simulink model "sudarshan_simulink3"  (R2021b)
settings: Solver=VariableStepAuto  StartTime=0.0  StopTime=0.01  RelTol=1e-3
settings Model: Creator=year2  LastModifiedBy=year2

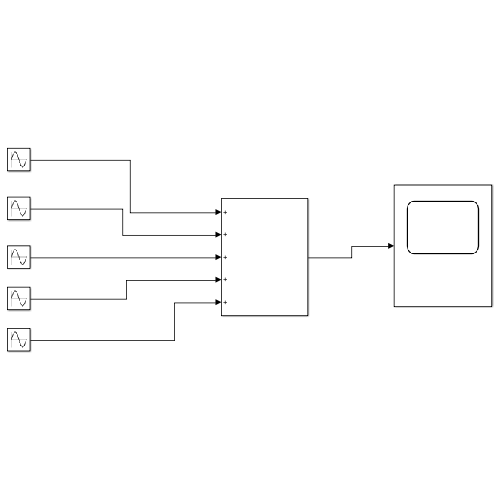
[thumbnail: Simulink's stored preview of the top-level diagram]
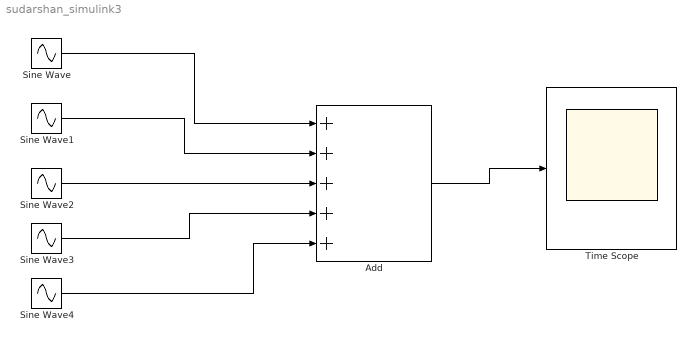
== system sudarshan_simulink3 ==
  Add : Sum  Inputs=+++++
  Sine Wave : Sin  Frequency=2*5*1000  SampleTime=0
  Sine Wave1 : Sin  Amplitude=1/3  Frequency=2*5*3000  SampleTime=0
  Sine Wave2 : Sin  Amplitude=1/5  Frequency=2*5*5000  SampleTime=0
  Sine Wave3 : Sin  Amplitude=1/7  Frequency=2*5*7000  SampleTime=0
  Sine Wave4 : Sin  Amplitude=1/9  Frequency=2*5*9000  SampleTime=0
  Time Scope : Scope
  wires:
  Add/1 -> Time Scope/1
  Sine Wave2/1 -> Add/3
  Sine Wave1/1 -> Add/2
  Sine Wave/1 -> Add/1
  Sine Wave3/1 -> Add/4
  Sine Wave4/1 -> Add/5
